simulink library "PEB601MSEREF"  (R2014b)
settings: Solver=ode45  StartTime=0.0  StopTime=10.0  RelTol=1e-3
libraries: PEPS101MSEREF x3
settings Model: Creator=vda2sh  LastModifiedBy=vda2sh

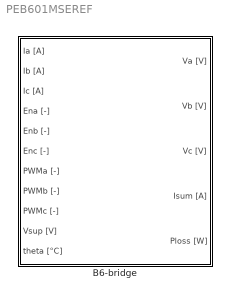
== system PEB601MSEREF ==
  B6-bridge : Subsystem  Tag=PEB601MSEREF  mask(PEB601MSEREF){RT20=1e-3, RD20=1e-3, VT20=0, VD20=0.7, IGBT=off, Ieps=1e-3, alphaRT=0, alphaRD=0, alphaVT=0, alphaVD=0}
      mask prompts: RT20 "Transistor on resistance at 20 °C [Ohm]"; RD20 "Diode on resistance at 20 °C [Ohm]"; VT20 "Transistor forward voltage at 20 °C [V]"; VD20 "Diode forward voltage at 20 °C [V]"; IGBT "Enable IGBT"; Ieps "Numerical parameter for diode treatment [A]"; alphaRT "Thermal coefficient of transistor on resistance [1/K]"; alphaRD "Thermal coefficient of diode on resistance [1/K]"; alphaVT "Thermal coefficient of transistor forward voltage [1/K]"; alphaVD "Thermal coefficient of diode forward voltage [1/K]"
      mask help:
      | PEB601MSEREF - B6-bridge
      |
      | This is a model of a B6-bridge - also denoted drive - with 6 switches, each switch consisting
      | of a transistor parallel connected to a free-wheel diode.
      | The 6 switches are allocated in three single power stages.
      settings: AttributesFormatString=<%<Tag>>
      mask Help: eval('show_docs_mseref_powerelectronics(''PEB601MSEREF'')')
      mask Callback IGBT:
      | % Defining temporary Matlab workspace structure variable `MCBVP__`
      | % `Mask Callback Variable ...` with following fields:
      | % `IGBT`: `0` if Enable IGBT is false, `1` if true
      | % `enables`: `on` if a parameter value can be changed in the mask, `off`
      | % otherwise
      | % `visibilities`: `on` if a parameter may be visible in the mask, `off`
      | % otherwise
      | 
      | % Comparing `IGBT` parameter value with `on`
      | MCBVP__.IGBT = strcmp(get_param(gcb,'IGBT'), 'on');
      | 
      | % Initializing `enables` and `visibilities` fields
      | MCBVP__.enables = {};
      | MCBVP__.visibilities = {};
      | 
      | % Setting `enables` and `visibilities` for `Transistor on resistance at
      | % 20°C`
      | MCBVP__.enables{end + 1} = 'on';
      | MCBVP__.visibilities{end + 1} = 'on';
      | 
      | % Setting `enables` and `visibilities` for `Diode on resistance at 20°C`
      | MCBVP__.enables{end + 1} = 'on';
      | MCBVP__.visibilities{end + 1} = 'on';
      | 
      | % Setting `enables` and `visibilities` for `Transistor forward voltage at 20°C`
      | if MCBVP__.IGBT==true
      |     MCBVP__.enables{end + 1} = 'on';
      |     MCBVP__.visibilities{end + 1} = 'on';
      | else
      |     MCBVP__.enables{end + 1} = 'off';
      |     MCBVP__.visibilities{end + 1} = 'off';
      | end
      | 
      | % Setting `enables` and `visibilities` for `Diode forward voltage at 20°C`
      | MCBVP__.enables{end + 1} = 'on';
      | MCBVP__.visibilities{end + 1} = 'on';
      | 
      | % Setting `enables` and `visibilities` for `Enable IGBT`
      | MCBVP__.enables{end + 1} = 'on';
      | MCBVP__.visibilities{end + 1} = 'on';
      | 
      | % Setting `enables` and `visibilities` for `Numerical parameter for diode treatment`
      | MCBVP__.enables{end + 1} = 'on';
      | MCBVP__.visibilities{end + 1} = 'on';
      | 
      | % Setting `enables` and `visibilities` for `Thermal coefficient of transistor on resistance`
      | MCBVP__.enables{end + 1} = 'on';
      | MCBVP__.visibilities{end + 1} = 'on';
      | 
      | % Setting `enables` and `visibilities` for `Thermal coefficient of diode on resistance`
      | MCBVP__.enables{end + 1} = 'on';
      | MCBVP__.visibilities{end + 1} = 'on';
      | 
      | % Setting `enables` and `visibilities` for `Thermal coefficient of transistor forward voltage`
      | if MCBVP__.IGBT==true
      |     MCBVP__.enables{end + 1} = 'on';
      |     MCBVP__.visibilities{end + 1} = 'on';
      | else
      |     MCBVP__.enables{end + 1} = 'off';
      |     MCBVP__.visibilities{end + 1} = 'off';
      | end
      | 
      | % Setting `enables` and `visibilities` for `Thermal coefficient of diode forward voltage`
      | MCBVP__.enables{end + 1} = 'on';
      | MCBVP__.visibilities{end + 1} = 'on';
      | 
      | % Setting `MaskEnables` and `MaskVisibilities` in current block
      | set_param(gcb, 'MaskEnables', MCBVP__.enables);
      | set_param(gcb, 'MaskVisibilities', MCBVP__.visibilities);
      | 
      | % Clear variable `MCBVP__`
      | clear MCBVP__;
      mask Display:
      | image(imread('PEB601MSEREF.png'),[0,0, 1,1])
      | text(0.6,0.15, 'MSE')
      | port_label('input',1,'Ia [A]')
      | port_label('input',2,'Ib [A]')
      | port_label('input',3,'Ic [A]')
      | port_label('input',4,'Ena [-]')
      | port_label('input',5,'Enb [-]')
      | port_label('input',6,'Enc [-]')
      | port_label('input',7,'PWMa [-]')
      | port_label('input',8,'PWMb [-]')
      | port_label('input',9,'PWMc [-]')
      | port_label('input',10,'Vsup [V]')
      | port_label('input',11,'theta [°C]')
      | port_label('output',1,'Va [V]')
      | port_label('output',2,'Vb [V]')
      | port_label('output',3,'Vc [V]')
      | port_label('output',4,'Isum [A]')
      | port_label('output',5,'Ploss [W]')

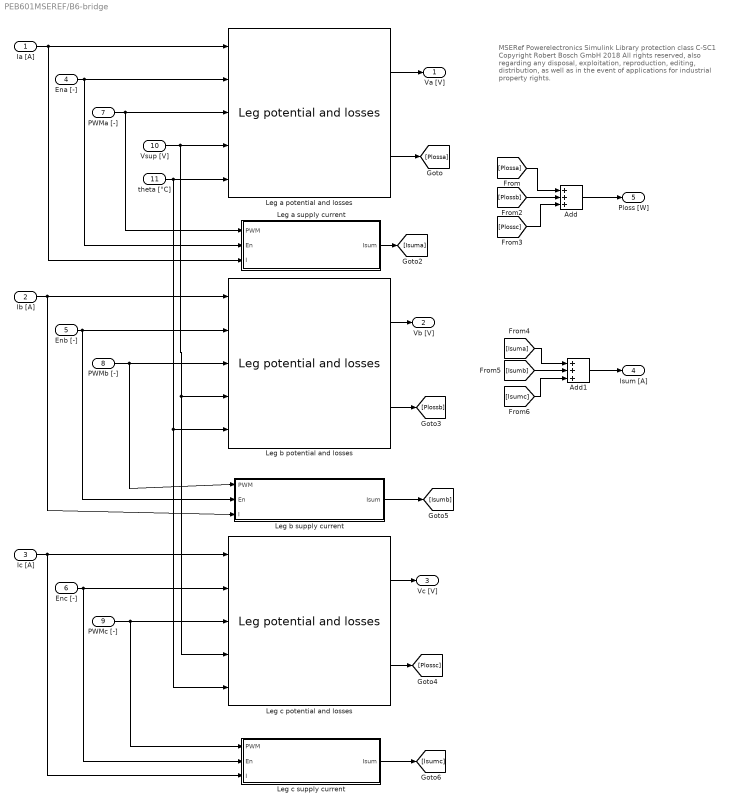
== system PEB601MSEREF/B6-bridge ==
  note: MSERef Powerelectronics Simulink Library
      | protection class C-SC1
      |
      | Copyright Robert Bosch GmbH 2018
      |
      | All rights reserved, also regarding any disposal, exploitation,
      | reproduction, editing, distribution, as well as in the event of
      | applications for industrial property rights.
  Ia [A] : Inport
  Ib [A] : Inport  Port=2
  Ic [A] : Inport  Port=3
  Ena [-] : Inport  Port=4
  Enb [-] : Inport  Port=5
  Enc [-] : Inport  Port=6
  PWMa [-] : Inport  Port=7
  PWMb [-] : Inport  Port=8
  PWMc [-] : Inport  Port=9
  Vsup [V] : Inport  Port=10
  theta [°C] : Inport  Port=11
  Add : Sum  Inputs=+++
  Add1 : Sum  Inputs=+++
  Leg a potential and losses : PEPS101MSEREF/Single power stage/Leg potential and losses  RT20=RT20  RD20=RD20  VT20=VT20  VD20=VD20  IGBT=IGBT  Ieps=Ieps  alphaRT=alphaRT  alphaRD=alphaRD  alphaVT=alphaVT  alphaVD=alphaVD
  Leg a supply current : MATLAB Function  TreatAsAtomicUnit=on
  Leg b potential and losses : PEPS101MSEREF/Single power stage/Leg potential and losses  RT20=RT20  RD20=RD20  VT20=VT20  VD20=VD20  IGBT=IGBT  Ieps=Ieps  alphaRT=alphaRT  alphaRD=alphaRD  alphaVT=alphaVT  alphaVD=alphaVD
  Leg b supply current : MATLAB Function  TreatAsAtomicUnit=on
  Leg c potential and losses : PEPS101MSEREF/Single power stage/Leg potential and losses  RT20=RT20  RD20=RD20  VT20=VT20  VD20=VD20  IGBT=IGBT  Ieps=Ieps  alphaRT=alphaRT  alphaRD=alphaRD  alphaVT=alphaVT  alphaVD=alphaVD
  Leg c supply current : MATLAB Function  TreatAsAtomicUnit=on
  Va [V] : Outport
  Vb [V] : Outport  Port=2
  Vc [V] : Outport  Port=3
  Isum [A] : Outport  Port=4
  Ploss [W] : Outport  Port=5
  wires:
  Leg a supply current/1(Isum) -> [Isuma]
  PWMa [-]/1 -> Leg a potential and losses/3, Leg a supply current/1(PWM)
  Ena [-]/1 -> Leg a potential and losses/2, Leg a supply current/2(En)
  Ia [A]/1 -> Leg a potential and losses/1, Leg a supply current/3(I)
  Leg b supply current/1(Isum) -> [Isumb]
  PWMb [-]/1 -> Leg b potential and losses/3, Leg b supply current/1(PWM)
  Enb [-]/1 -> Leg b potential and losses/2, Leg b supply current/2(En)
  Ib [A]/1 -> Leg b potential and losses/1, Leg b supply current/3(I)
  Leg c supply current/1(Isum) -> [Isumc]
  theta [°C]/1 -> Leg a potential and losses/5, Leg c potential and losses/5, Leg b potential and losses/5
  Vsup [V]/1 -> Leg a potential and losses/4, Leg c potential and losses/4, Leg b potential and losses/4
  PWMc [-]/1 -> Leg c potential and losses/3, Leg c supply current/1(PWM)
  Enc [-]/1 -> Leg c potential and losses/2, Leg c supply current/2(En)
  Ic [A]/1 -> Leg c potential and losses/1, Leg c supply current/3(I)
  Leg a potential and losses/1 -> Va [V]/1
  Leg b potential and losses/1 -> Vb [V]/1
  Leg c potential and losses/1 -> Vc [V]/1
  Leg a potential and losses/2 -> [Plossa]
  Leg b potential and losses/2 -> [Plossb]
  Leg c potential and losses/2 -> [Plossc]
  [Plossa] -> Add/1
  [Plossb] -> Add/2
  [Plossc] -> Add/3
  Add/1 -> Ploss [W]/1
  [Isuma] -> Add1/1
  [Isumb] -> Add1/2
  [Isumc] -> Add1/3
  Add1/1 -> Isum [A]/1

== matlab function PEB601MSEREF/B6-bridge/Leg a supply current ==
  data: PWM input; Isum output; En input; I input
function Isum = PEPS101MSEREF_supply_current(PWM,En,I)
% This function is used to compute the supply current.
%
%  MSERef Powerelectronics Simulink Library 
%  protection class C-SC1
%
%  Copyright Robert Bosch GmbH 2018
%
%  All rights reserved, also regarding any disposal, exploitation,
%  reproduction, editing, distribution, as well as in the event of
%  applications for industrial property rights.

if ( En >= 0.5 ) % Implementing equation (3) from the `PEPS101MSEREF_details` documentation
    Isum = I*PWM;
else % ( En < 0.5 ) % Implementing equation (4) from the `PEPS101MSEREF_details` documentation
    Isum = min(I,0);
end

== matlab function PEB601MSEREF/B6-bridge/Leg b supply current ==
  data: PWM input; Isum output; En input; I input
function Isum = PEPS101MSEREF_supply_current(PWM,En,I)
% This function is used to compute the supply current.
%
%  MSERef Powerelectronics Simulink Library 
%  protection class C-SC1
%
%  Copyright Robert Bosch GmbH 2018
%
%  All rights reserved, also regarding any disposal, exploitation,
%  reproduction, editing, distribution, as well as in the event of
%  applications for industrial property rights.

if ( En >= 0.5 ) % Implementing equation (3) from the `PEPS101MSEREF_details` documentation
    Isum = I*PWM;
else % ( En < 0.5 ) % Implementing equation (4) from the `PEPS101MSEREF_details` documentation
    Isum = min(I,0);
end

== matlab function PEB601MSEREF/B6-bridge/Leg c supply current ==
  data: PWM input; Isum output; En input; I input
function Isum = PEPS101MSEREF_supply_current(PWM,En,I)
% This function is used to compute the supply current.
%
%  MSERef Powerelectronics Simulink Library 
%  protection class C-SC1
%
%  Copyright Robert Bosch GmbH 2018
%
%  All rights reserved, also regarding any disposal, exploitation,
%  reproduction, editing, distribution, as well as in the event of
%  applications for industrial property rights.

if ( En >= 0.5 ) % Implementing equation (3) from the `PEPS101MSEREF_details` documentation
    Isum = I*PWM;
else % ( En < 0.5 ) % Implementing equation (4) from the `PEPS101MSEREF_details` documentation
    Isum = min(I,0);
end
